simulink model "h2omnix_heading_vis"  (R2022b)
settings: Solver=ode4  StartTime=0.0  StopTime=inf  FixedStep=0.05  RelTol=1e-3
values from neighbouring files (symbols this model uses):
  nu_max = [0.5,0.5,1]'    [parameters.m]
  nu_min = -nu_max    [parameters.m]
  pcKd = pcKd.*disable    [parameters.m]
  pcKp = pcKp.*disable    [parameters.m]
  vcKi = vcKi.*disable    [parameters.m]
  vcKp = vcKp.*disable    [parameters.m]
  vcKt = vcKt.*disable    [parameters.m]
  wn = 3*wpn/2    [parameters.m]
  wpn = [1.2, 1.2, 1]'    [parameters.m]
libraries: MarineRoboticsLib x2, MarineRoboticsLibEx x1, matrix_library x1, simulink x1
settings Model: DataDictionary=ros2lib.sldd  Creator=dnad  LastModifiedBy=dnad

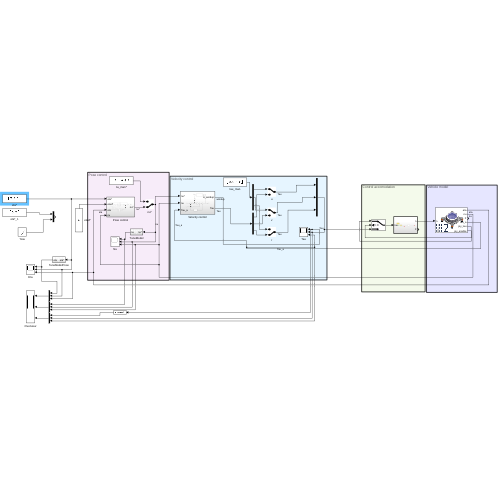
[thumbnail: Simulink's stored preview of the top-level diagram]
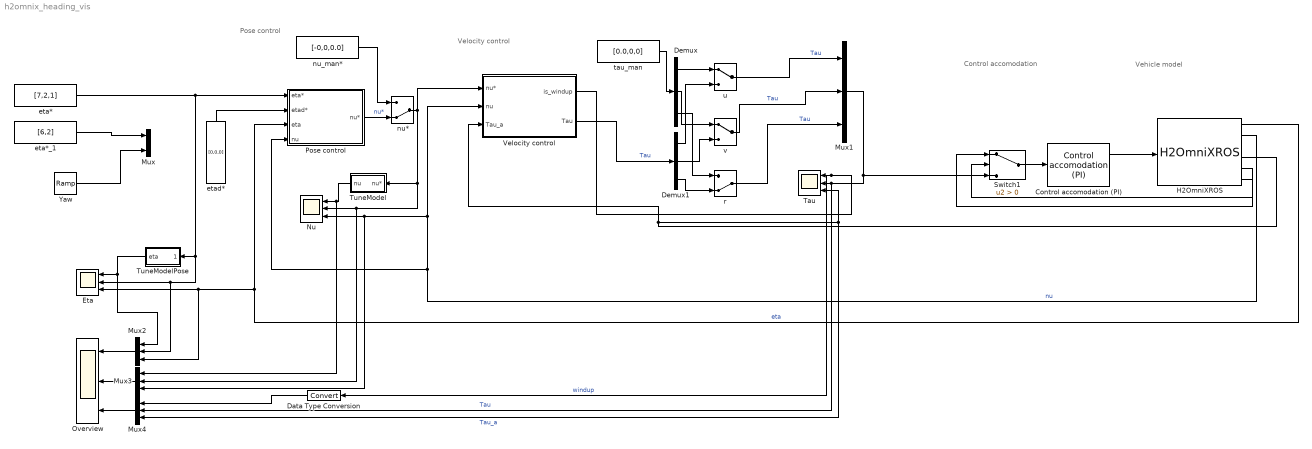
== system h2omnix_heading_vis ==
  note: Control accomodation
  note: Vehicle model
  note: Pose control
  note: Velocity control
  Control accomodation (PI) : MarineRoboticsLibEx/Control accomodation (PI)  SystemSampleTime=-1  VariantActivationTime=update diagram  Latency=0  AutoFrameSizeCalculation=off
  Data Type Conversion : DataTypeConversion  SaturateOnIntegerOverflow=off  RndMeth=Floor
  Demux : Demux  Outputs=3
  Demux1 : Demux  Outputs=3
  Eta : Scope  NumInputPorts=3
  H2OmniXROS : MarineRoboticsLib/H2OmniXROS  vehicle_name=vis  max_pwm=0.4  pwm_topic=/vis/pwm_out  joy_topic=/vis/joy  odometry_topic=/vis/odometry/filtered
  Mux : Mux  Inputs=2
  Mux{1..4} (4 alike) : Mux  Inputs=3
  Nu : Scope  NumInputPorts=3
  Overview : Scope  NumInputPorts=3
  Pose control : Subsystem
  Switch1 : Switch  Criteria=u2 > Threshold  SaturateOnIntegerOverflow=off  InputSameDT=off
  Tau : Scope  NumInputPorts=3
  TuneModel : Subsystem
  TuneModelPose : Subsystem
  Velocity control : Subsystem
  Yaw : simulink/Sources/Ramp  slope=0.5  start=0  InitialOutput=0
  eta* : Constant  Value=[7,2,1]
  eta*_1 : Constant  Value=[6,2]
  etad* : Constant  Value=[0,0,0]
  nu* : ManualSwitch  CurrentSetting=0
  nu_man* : Constant  Value=[-0,0,0.0]
  r : ManualSwitch  CurrentSetting=0
  tau_man : Constant  Value=[0.0,0,0]
  u : ManualSwitch
  v : ManualSwitch
  wires:
  Switch1/1 -> Control accomodation (PI)/1
  Control accomodation (PI)/1 -> H2OmniXROS/1
  H2OmniXROS/5 -> Switch1/1
  H2OmniXROS/6 -> Switch1/2
  TuneModelPose/1(eta) -> Mux2/1, Eta/1
  Velocity control/1(is_windup) -> Data Type Conversion/1, Tau/1  "windup"
  etad*/1 -> Pose control/2(etad*)
  Pose control/1(nu*) -> nu*/2  "nu*"
  eta*_1/1 -> Mux/1
  Mux1/1 -> Mux4/2, Tau/2, Switch1/3  "Tau"
  TuneModel/1(nu) -> Mux3/1, Nu/1
  nu_man*/1 -> nu*/1
  H2OmniXROS/1 -> Pose control/3(eta), Mux2/3, Eta/3  "eta"
  H2OmniXROS/2 -> Velocity control/2(nu), Mux3/3, Nu/3, Pose control/4(nu)  "nu"
  H2OmniXROS/4 -> Velocity control/3(Tau_a), Mux4/3, Tau/3  "Tau_a"
  Yaw/1 -> Mux/2
  nu*/1 -> Mux3/2, Nu/2, TuneModel/1(nu*), Velocity control/1(nu*)
  eta*/1 -> Mux2/2, Eta/2, TuneModelPose/1(eta*), Pose control/1(eta*)
  tau_man/1 -> Demux/1
  Velocity control/2(Tau) -> Demux1/1  "Tau"
  Demux/1 -> u/1
  Demux1/1 -> u/2
  Demux/2 -> v/1
  Demux1/2 -> v/2
  Demux/3 -> r/1
  Demux1/3 -> r/2
  r/1 -> Mux1/3  "Tau"
  v/1 -> Mux1/2  "Tau"
  u/1 -> Mux1/1  "Tau"
  Mux2/1 -> Overview/1
  Mux3/1 -> Overview/2
  Mux4/1 -> Overview/3
  Data Type Conversion/1 -> Mux4/1

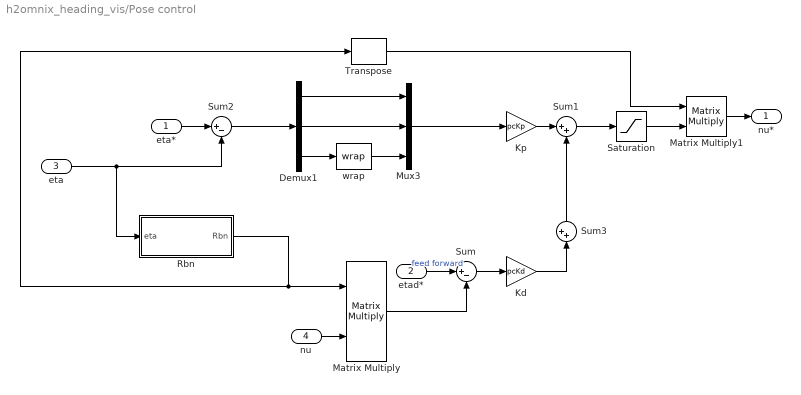
== system h2omnix_heading_vis/Pose control ==
  eta* : Inport
  etad* : Inport  Port=2
  eta : Inport  Port=3
  nu : Inport  Port=4
  Demux1 : Demux  Outputs=3
  Kd : Gain  Gain=pcKd
  Kp : Gain  Gain=pcKp
  Matrix Multiply : Product  Multiplication=Matrix(*)
  Matrix Multiply1 : Product  Multiplication=Matrix(*)
  Mux3 : Mux  Inputs=3
  Rbn : MATLAB Function  TreatAsAtomicUnit=on
  Saturation : Saturate  UpperLimit=nu_max  LowerLimit=nu_min
  Sum : Sum  Inputs=|+-
  Sum1 : Sum  Inputs=|++
  Sum2 : Sum  Inputs=|+-
  Sum3 : Sum  Inputs=++|
  Transpose : matrix_library/Transpose
  wrap : MarineRoboticsLib/wrap  SystemSampleTime=-1  VariantActivationTime=update diagram  Latency=0  AutoFrameSizeCalculation=off
      settings: LibrarySourceBlock=|
      | simulink/User-Defined
      | Functions/MATLAB Function
  nu* : Outport
  wires:
  Sum/1 -> Kd/1
  eta/1 -> Rbn/1(eta), Sum2/2
  etad*/1 -> Sum/1  "feed forward"
  Kp/1 -> Sum1/1
  eta*/1 -> Sum2/1
  Sum2/1 -> Demux1/1
  Demux1/1 -> Mux3/1
  Demux1/2 -> Mux3/2
  Demux1/3 -> wrap/1
  wrap/1 -> Mux3/3
  Mux3/1 -> Kp/1
  Sum1/1 -> Saturation/1
  Sum3/1 -> Sum1/2
  Kd/1 -> Sum3/2
  Rbn/1(Rbn) -> Matrix Multiply/1, Transpose/1
  Matrix Multiply1/1 -> nu*/1
  nu/1 -> Matrix Multiply/2
  Matrix Multiply/1 -> Sum/2
  Saturation/1 -> Matrix Multiply1/2
  Transpose/1 -> Matrix Multiply1/1

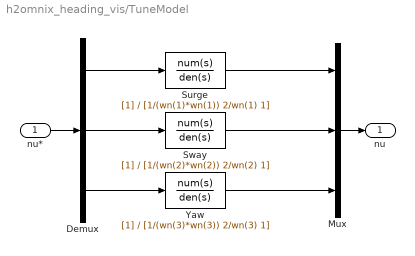
== system h2omnix_heading_vis/TuneModel ==
  nu* : Inport
  Demux : Demux  Outputs=3
  Mux : Mux  Inputs=3
  Surge : TransferFcn  Denominator=[1/(wn(1)*wn(1)) 2/wn(1) 1]
  Sway : TransferFcn  Denominator=[1/(wn(2)*wn(2)) 2/wn(2) 1]
  Yaw : TransferFcn  Denominator=[1/(wn(3)*wn(3)) 2/wn(3) 1]
  nu : Outport
  wires:
  nu*/1 -> Demux/1
  Demux/1 -> Surge/1
  Surge/1 -> Mux/1
  Mux/1 -> nu/1
  Sway/1 -> Mux/2
  Demux/2 -> Sway/1
  Demux/3 -> Yaw/1
  Yaw/1 -> Mux/3

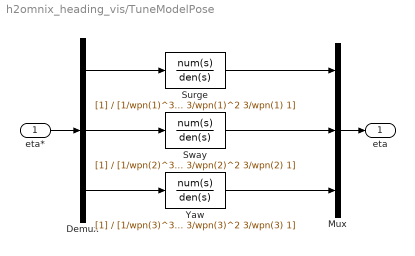
== system h2omnix_heading_vis/TuneModelPose ==
  eta* : Inport
  Demux : Demux  Outputs=3
  Mux : Mux  Inputs=3
  Surge : TransferFcn  Denominator=[1/wpn(1)^3 3/wpn(1)^2 3/wpn(1) 1]
  Sway : TransferFcn  Denominator=[1/wpn(2)^3 3/wpn(2)^2 3/wpn(2) 1]
  Yaw : TransferFcn  Denominator=[1/wpn(3)^3 3/wpn(3)^2 3/wpn(3) 1]
  eta : Outport
  wires:
  eta*/1 -> Demux/1
  Demux/1 -> Surge/1
  Surge/1 -> Mux/1
  Mux/1 -> eta/1
  Sway/1 -> Mux/2
  Demux/2 -> Sway/1
  Demux/3 -> Yaw/1
  Yaw/1 -> Mux/3

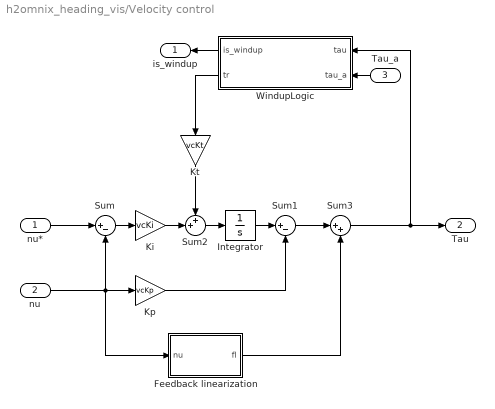
== system h2omnix_heading_vis/Velocity control ==
  nu* : Inport
  nu : Inport  Port=2
  Tau_a : Inport  Port=3
  Feedback linearization : MATLAB Function  TreatAsAtomicUnit=on
  Integrator : Integrator
  Ki : Gain  Gain=vcKi
  Kp : Gain  Gain=vcKp
  Kt : Gain  Gain=vcKt
  Sum : Sum  Inputs=|+-
  Sum1 : Sum  Inputs=|+-
  Sum2 : Sum  Inputs=++|
  Sum3 : Sum  Inputs=|++
  WindupLogic : MATLAB Function  TreatAsAtomicUnit=on
  is_windup : Outport
  Tau : Outport  Port=2
  wires:
  Tau_a/1 -> WindupLogic/2(tau_a)
  nu/1 -> Feedback linearization/1(nu), Kp/1, Sum/2
  Integrator/1 -> Sum1/1
  nu*/1 -> Sum/1
  Sum/1 -> Ki/1
  Sum2/1 -> Integrator/1
  Kp/1 -> Sum1/2
  Ki/1 -> Sum2/2
  WindupLogic/1(is_windup) -> is_windup/1
  WindupLogic/2(tr) -> Kt/1
  Sum1/1 -> Sum3/1
  Sum3/1 -> WindupLogic/1(tau), Tau/1
  Feedback linearization/1(fl) -> Sum3/2
  Kt/1 -> Sum2/1

== matlab function h2omnix_heading_vis/Velocity control/WindupLogic ==
  data: tau input; is_windup output; tau_a input; tr output
function [is_windup, tr] = checkWindup(tau, tau_a)
% Consider the tracking within tolerances
tol = 0.01;
is_windup = abs(tau-tau_a)>tol & abs(tau)>0.1;
tr = is_windup.*(tau_a - tau);
end

== matlab function h2omnix_heading_vis/Pose control/Rbn ==
  data: eta input; Rbn output
function Rbn = RotMatrix(eta)

cp = cos(eta(3));
sp = sin(eta(3));

Rbn = [cp -sp 0;
     sp  cp 0;
      0   0 1];

== matlab function h2omnix_heading_vis/Velocity control/Feedback linearization ==
  data: nu input; fl output
function fl = feedback_lin(nu)
Betaa = [0, 0, 0]';
fl = Betaa.*abs(nu).*nu;
end
